simulink model "Bandstop_4th"  (R2017b)
settings: Solver=VariableStepAuto  StartTime=0.0  StopTime=1  RelTol=1e-3
undefined symbols (not defined in the file or in its folder): a, Afixed, b, Bfixed
libraries: dsparch4 x1, modelsimlib x1
settings Model: Creator=sonic  LastModifiedBy=sonic

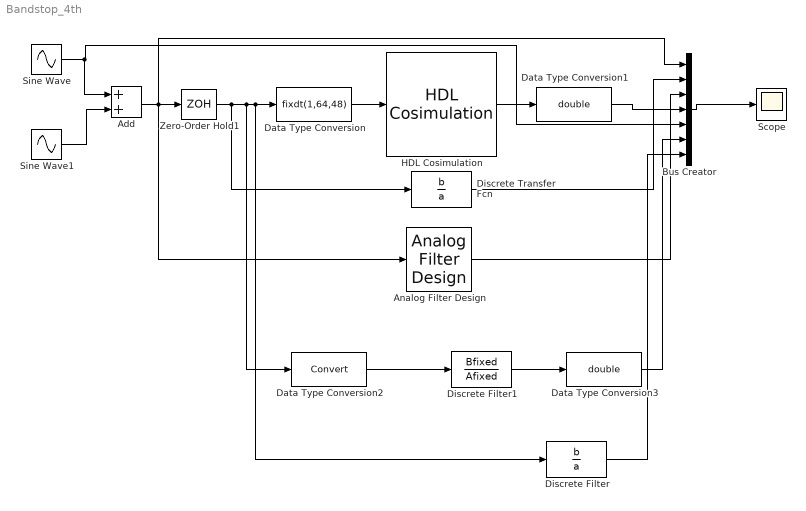
== system Bandstop_4th ==
  Add : Sum
  Analog Filter Design : dsparch4/Analog Filter Design  method=Elliptic  filttype=Bandpass  N=6  Wlo=1256  Whi=125663  Rp=1  Rs=30
  Bus Creator : BusCreator  Inputs=7
  Data Type Conversion : DataTypeConversion  OutDataTypeStr=fixdt(1,64,48)
  Data Type Conversion1 : DataTypeConversion  OutDataTypeStr=double
  Data Type Conversion2 : DataTypeConversion
  Data Type Conversion3 : DataTypeConversion  OutDataTypeStr=double
  Discrete Transfer Fcn : DiscreteTransferFcn  Numerator=b  Denominator=a  SampleTime=0.00002  NumCoefDataTypeStr=int16  DenCoefDataTypeStr=int16
  Discrete Filter : DiscreteFilter  Numerator=b  Denominator=a  SampleTime=0.00002
  Discrete Filter1 : DiscreteFilter  Numerator=Bfixed  Denominator=Afixed  SampleTime=0.00002  StateDataTypeStr=fixdt(1,64,48)  NumCoefDataTypeStr=fixdt(1,64,48)  DenCoefDataTypeStr=fixdt(1,64,48)  NumProductDataTypeStr=fixdt(1,64,48)  DenProductDataTypeStr=fixdt(1,64,48)  NumAccumDataTypeStr=fixdt(1,64,48)  DenAccumDataTypeStr=fixdt(1,64,48)  OutDataTypeStr=fixdt(1,64,48)
  HDL Cosimulation : modelsimlib/HDL Cosimulation  PortPaths=/elliptic_bandpass_filter/XIN;/elliptic_bandpass_filter/YOUT  PortModes=[1 2 ]  PortTimes=[-1,0.00002]  PortSigns=[-1 1 ]  PortFracLengths=[0,48]  CommLocal=on  CommSharedMemory=on  CommPortNumber=4449  CommShowInfo=on  ClockModes=[]  ClockTimes=[]  TclPreSimCommand="puts \"Running Simulink Cosimulation block.\""  TclPostSimCommand="puts \"done\""  TimingMode=s  TimingScaleFactor=1  idxCellArray={'UNUSED_VAR'}  CosimBypass=Full Simulation  AllowDirectFeedthrough=on  ProductName=EDA Simulator Link MQ  RunAutoTimescale=off  HdlClocks=0  PreRunTime=0  PreRunTimeUnit=ns
      settings: SourceProductName=HDL Verifier
  Scope : Scope
  Sine Wave : Sin  Amplitude=10  Frequency=12566  SampleTime=0
  Sine Wave1 : Sin  Amplitude=5  Frequency=157079  SampleTime=0
  Zero-Order Hold1 : ZeroOrderHold  SampleTime=0.00002
  wires:
  Sine Wave/1 -> Add/1, Bus Creator/5
  Sine Wave1/1 -> Add/2
  Add/1 -> Bus Creator/1, Analog Filter Design/1, Zero-Order Hold1/1
  Zero-Order Hold1/1 -> Data Type Conversion2/1, Discrete Filter/1, Data Type Conversion/1, Discrete Transfer Fcn/1
  Bus Creator/1 -> Scope/1
  Discrete Transfer Fcn/1 -> Bus Creator/2
  Analog Filter Design/1 -> Bus Creator/3
  Data Type Conversion1/1 -> Bus Creator/4
  Data Type Conversion/1 -> HDL Cosimulation/1
  HDL Cosimulation/1 -> Data Type Conversion1/1
  Data Type Conversion2/1 -> Discrete Filter1/1
  Discrete Filter1/1 -> Data Type Conversion3/1
  Data Type Conversion3/1 -> Bus Creator/6
  Discrete Filter/1 -> Bus Creator/7
